simulink model "nominal_REALTIME"  (R2020b)
settings: Solver=FixedStepDiscrete  StartTime=0.0  StopTime=10.0  FixedStep=0.01  RelTol=1e-3  EnableMultiTasking=on
values from neighbouring files (symbols this model uses):
  denHw = [0.03 0 0 0]    [data_v2_500.mat]    (also in data_v6_nominaldrift500.mat)
  denLPFz = [1 -0.978482055734]    [data_v2_500.mat]    (also in data_v6_nominaldrift500.mat)
  drv =     [data_v2_500.mat]    (also in data_v6_nominaldrift500.mat)
  gbox =     [data_v2_500.mat]    (also in data_v6_nominaldrift500.mat)
  N_u = 0    [data_v2_500.mat]    (also in data_v6_nominaldrift500.mat)
  N_x = [1 0 0 0]    [data_v2_500.mat]    (also in data_v6_nominaldrift500.mat)
  numHw = [1 0 0 -1]    [data_v2_500.mat]    (also in data_v6_nominaldrift500.mat)
  numLPFz = [0.0215179442657 0]    [data_v2_500.mat]    (also in data_v6_nominaldrift500.mat)
  sens =     [data_v2_500.mat]    (also in data_v6_nominaldrift500.mat)
  Ts = 0.01    [data_v2_500.mat]    (also in data_v6_nominaldrift500.mat)
  wheel =     [data_v2_500.mat]    (also in data_v6_nominaldrift500.mat)
undefined symbols (not defined in the file or in its folder): C_gain, DiscIntNeverNeededParam, T
libraries: BalRobTbx_baselib x9
settings Model: SILPILModeSetting=veronly  ExtModeTrigDuration=2  Creator=utente  LastModifiedBy=saviangiul
settings OptimizationCC: EnhancedBackFolding=on  PassReuseOutputArgsAs=Individual arguments  ZeroExternalMemoryAtStartup=off  ZeroInternalMemoryAtStartup=off  MaxStackSize=64  OptimizeBlockOrder=speed  DifferentSizesBufferReuse=on  OptimizationCustomize=off  EfficientTunableParamExpr=on
settings DebuggingCC: ParameterTunabilityLossMsg=error
settings HardwareCC: ProdBitPerInt=16  ProdBitPerPointer=16  ProdBitPerSizeT=16  ProdBitPerPtrDiffT=16  ProdLargestAtomicFloat=None  ProdWordSize=8  ProdHWDeviceType=Atmel->AVR
settings SFSimCC: MATLABDynamicMemAlloc=off
settings RTWCC: Description=Embedded Coder  SystemTargetFile=ert.tlc  HardwareBoard=Arduino Mega 2560  TemplateMakefile=ert_default_tmf  Toolchain=Arduino AVR  BuildConfiguration=Faster Runs
settings CodeAppCC: ForceParamTrailComments=on  IgnoreCustomStorageClasses=off  OperatorAnnotations=on  SimulinkDataObjDesc=on  SFDataObjDesc=on  InsertBlockDesc=on
settings ERTTargetCC: SupportContinuousTime=on  SupportVariableSizeSignals=on  ExtModeStaticAllocSize=2048

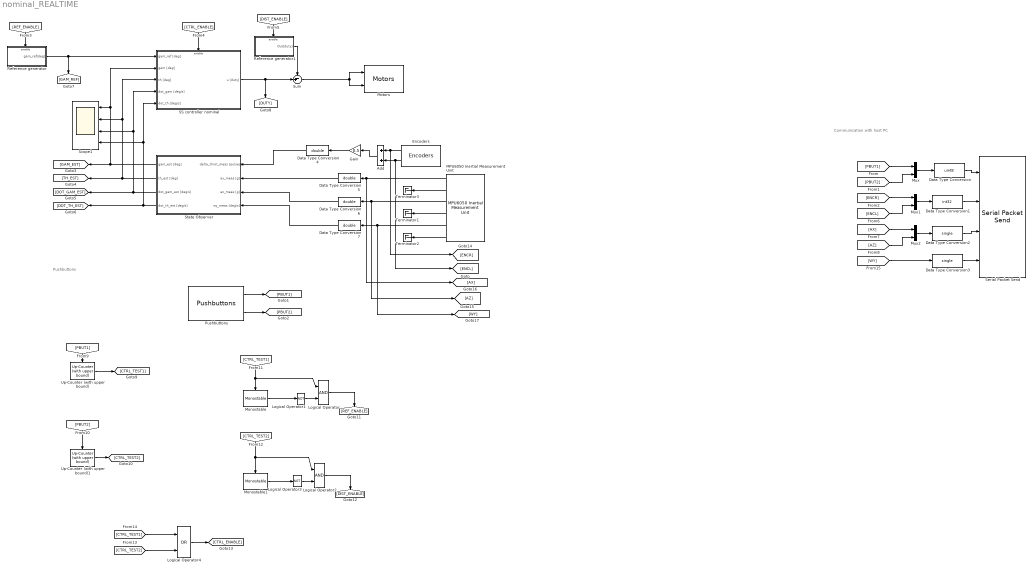
== system nominal_REALTIME ==
  note: Communication with host PC
  note: Pushbuttons
  Add : Sum
  Data Type Conversion : DataTypeConversion  OutDataTypeStr=uint8
  Data Type Conversion1 : DataTypeConversion  OutDataTypeStr=int32
  Data Type Conversion2 : DataTypeConversion  OutDataTypeStr=single
  Data Type Conversion3 : DataTypeConversion  OutDataTypeStr=single
  Data Type Conversion{4..7} (4 alike) : DataTypeConversion  OutDataTypeStr=double
  Encoders : BalRobTbx_baselib/Inputs/Encoders
      settings: SourceProductName=Balancing Robot Toolbox
  Gain : Gain  Gain=0.5
  Logical Operator : Logic  AllPortsSameDT=off  OutDataTypeStr=boolean
  Logical Operator1 : Logic  Operator=NOT  Inputs=1  AllPortsSameDT=off  OutDataTypeStr=boolean
  Logical Operator2 : Logic  AllPortsSameDT=off  OutDataTypeStr=boolean
  Logical Operator3 : Logic  Operator=NOT  Inputs=1  AllPortsSameDT=off  OutDataTypeStr=boolean
  Logical Operator4 : Logic  Operator=OR  AllPortsSameDT=off  OutDataTypeStr=boolean
  MPU6050 Inertial Measurement Unit : BalRobTbx_baselib/Inputs/MPU6050 Inertial Measurement Unit
      settings: SourceProductName=Balancing Robot Toolbox
  Monostable : BalRobTbx_baselib/Utilities/Monostable  Tp=1
      settings: SourceProductName=Balancing Robot Toolbox
  Monostable1 : BalRobTbx_baselib/Utilities/Monostable  Tp=1
      settings: SourceProductName=Balancing Robot Toolbox
  Motors : BalRobTbx_baselib/Outputs/Motors
      settings: SourceProductName=Balancing Robot Toolbox
  Mux : Mux  Inputs=2
  Mux1 : Mux  Inputs=2
  Mux2 : Mux  Inputs=2
  Pushbuttons : BalRobTbx_baselib/Inputs/Pushbuttons
      settings: SourceProductName=Balancing Robot Toolbox
  Reference generator : Subsystem
  Reference generator1 : Subsystem
  SS controller nominal : Subsystem
  Scope1 : Scope  NumInputPorts=4
  Serial Packet Send : BalRobTbx_baselib/Communication/Serial Packet Send  serialLinkOpt=Bluetooth  baudRateOpt=38400  waitHostTxCmd=on  txStartCmd=65  txStopCmd=66  packetSpec={'2*uint8', '2*int32', '2*single', 'single'}  cobsEncoded=on  nullTerminated=on  showEnablePort=off
      settings: SourceProductName=Balancing Robot Toolbox
  State Observer : Subsystem
  Sum : Sum  Inputs=-+|
  Terminator1 : Terminator
  Terminator2 : Terminator
  Terminator3 : Terminator
  Up-Counter (with upper bound) : BalRobTbx_baselib/Utilities/Up-Counter (with upper bound)  CMAX=10  C0=0
      settings: SourceProductName=Balancing Robot Toolbox
  Up-Counter (with upper bound)1 : BalRobTbx_baselib/Utilities/Up-Counter (with upper bound)  CMAX=10  C0=0
      settings: SourceProductName=Balancing Robot Toolbox
  wires:
  Reference generator/1(gam_ref[deg]) -> [GAM_REF], SS controller nominal/1(gam_ref [deg])
  Data Type Conversion4/1 -> State Observer/1("delta_throt_meas [pulses] ")
  State Observer/2(th_est [deg]) -> [TH_EST], SS controller nominal/3(th [deg]), Scope1/2
  Data Type Conversion6/1 -> State Observer/3("az_meas [g] ")
  Reference generator1/1(Out[duty]) -> Sum/1
  State Observer/1(gam_est [deg]) -> [GAM_EST], SS controller nominal/2(gam [deg]), Scope1/1
  SS controller nominal/1(u [duty]) -> [DUTY], Sum/2
  State Observer/4(dot_th_est [deg/s]) -> [DOT_TH_EST], SS controller nominal/5(dot_th [deg/s]), Scope1/4
  State Observer/3(dot_gam_est [deg/s]) -> [DOT_GAM_EST], SS controller nominal/4(dot_gam [deg/s]), Scope1/3
  Data Type Conversion7/1 -> State Observer/4(wy_meas [deg/s])
  [REF_ENABLE] -> Reference generator/Enable
  [CTRL_ENABLE] -> SS controller nominal/Enable
  [DIST_ENABLE] -> Reference generator1/Enable
  [CTRL_TEST1] -> Monostable/Enable, Logical Operator/1
  Logical Operator/1 -> [REF_ENABLE]
  Logical Operator1/1 -> Logical Operator/2
  Logical Operator3/1 -> Logical Operator2/2
  Logical Operator2/1 -> [DIST_ENABLE]
  [CTRL_TEST2] -> Logical Operator2/1, Monostable1/Enable
  [CTRL_TEST1] -> Logical Operator4/1
  [CTRL_TEST2] -> Logical Operator4/2
  Logical Operator4/1 -> [CTRL_ENABLE]
  Sum/1 -> Motors/2, Motors/1
  Pushbuttons/1 -> [PBUT1]
  Pushbuttons/2 -> [PBUT2]
  Monostable/1 -> Logical Operator1/1
  Monostable1/1 -> Logical Operator3/1
  Up-Counter (with upper bound)1/1 -> [CTRL_TEST2]
  [PBUT2] -> Up-Counter (with upper bound)1/Trigger
  [PBUT1] -> Up-Counter (with upper bound)/Trigger
  Up-Counter (with upper bound)/1 -> [CTRL_TEST1]
  [PBUT1] -> Mux/1
  [PBUT2] -> Mux/2
  [ENCR] -> Mux1/1
  [ENCL] -> Mux1/2
  [AX] -> Mux2/1
  [AZ] -> Mux2/2
  [WY] -> Data Type Conversion3/1
  Data Type Conversion3/1 -> Serial Packet Send/4
  Mux2/1 -> Data Type Conversion2/1
  Data Type Conversion2/1 -> Serial Packet Send/3
  Mux1/1 -> Data Type Conversion1/1
  Data Type Conversion1/1 -> Serial Packet Send/2
  Mux/1 -> Data Type Conversion/1
  Data Type Conversion/1 -> Serial Packet Send/1
  Encoders/2 -> Add/2, [ENCL]
  Gain/1 -> Data Type Conversion4/1
  MPU6050 Inertial Measurement Unit/3 -> [AZ], Data Type Conversion6/1
  MPU6050 Inertial Measurement Unit/5 -> [WY], Data Type Conversion7/1
  MPU6050 Inertial Measurement Unit/4 -> Terminator1/1
  Encoders/1 -> [ENCR], Add/1
  Add/1 -> Gain/1
  MPU6050 Inertial Measurement Unit/1 -> [AX], Data Type Conversion5/1
  MPU6050 Inertial Measurement Unit/2 -> Terminator3/1
  MPU6050 Inertial Measurement Unit/6 -> Terminator2/1
  Data Type Conversion5/1 -> State Observer/2("ax_meas [g] ")

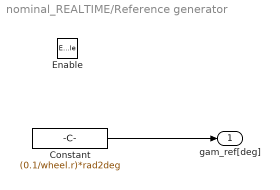
== system nominal_REALTIME/Reference generator ==
  Enable : EnablePort  StatesWhenEnabling=reset
  Constant : Constant  Value=(0.1/wheel.r)*rad2deg  SampleTime=0.01
  gam_ref[deg] : Outport  InitialOutput=[0]
  wires:
  Constant/1 -> gam_ref[deg]/1

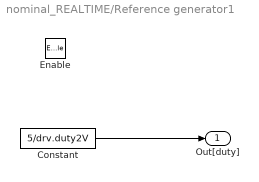
== system nominal_REALTIME/Reference generator1 ==
  Enable : EnablePort  StatesWhenEnabling=reset
  Constant : Constant  Value=5/drv.duty2V  SampleTime=0.01
  Out[duty] : Outport  InitialOutput=[0]
  wires:
  Constant/1 -> Out[duty]/1

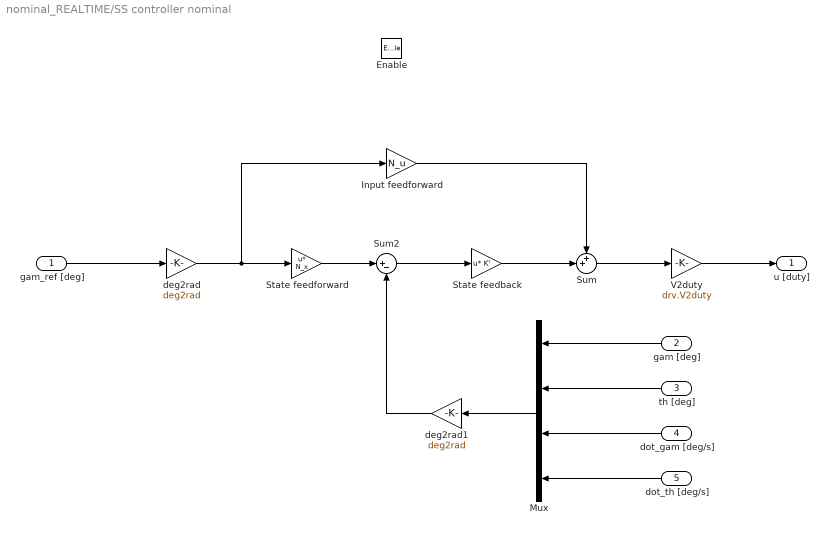
== system nominal_REALTIME/SS controller nominal ==
  gam_ref [deg] : Inport
  gam [deg] : Inport  Port=2
  th [deg] : Inport  Port=3
  dot_gam [deg/s] : Inport  Port=4
  dot_th [deg/s] : Inport  Port=5
  Enable : EnablePort  StatesWhenEnabling=reset
  Input feedforward : Gain  Gain=N_u
  Mux : Mux
  State feedback : Gain  Gain=K'  Multiplication=Matrix(u*K)
  "State feedforward\t" : Gain  Gain=N_x  Multiplication=Matrix(u*K)
  Sum : Sum  Inputs=++|
  Sum2 : Sum  Inputs=|+-
  V2duty : Gain  Gain=drv.V2duty
  deg2rad : Gain  Gain=deg2rad
  deg2rad1 : Gain  Gain=deg2rad
  u [duty] : Outport  InitialOutput=[0]
  wires:
  gam_ref [deg]/1 -> deg2rad/1
  deg2rad/1 -> Input feedforward/1, "State feedforward\t"/1
  State feedback/1 -> Sum/2
  "State feedforward\t"/1 -> Sum2/1
  Sum2/1 -> State feedback/1
  Input feedforward/1 -> Sum/1
  Sum/1 -> V2duty/1
  V2duty/1 -> u [duty]/1
  gam [deg]/1 -> Mux/1
  Mux/1 -> deg2rad1/1
  dot_gam [deg/s]/1 -> Mux/3
  th [deg]/1 -> Mux/2
  dot_th [deg/s]/1 -> Mux/4
  deg2rad1/1 -> Sum2/2

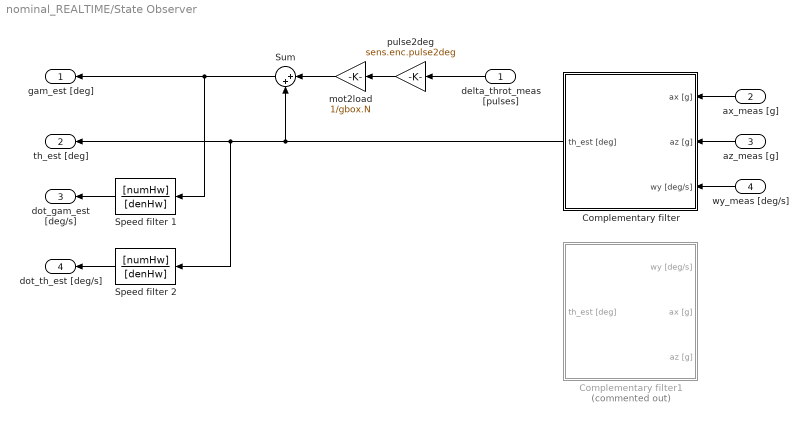
== system nominal_REALTIME/State Observer ==
  "delta_throt_meas [pulses] " : Inport
  "ax_meas [g] " : Inport  Port=2
  "az_meas [g] " : Inport  Port=3
  wy_meas [deg/s] : Inport  Port=4
  Complementary filter : Subsystem
  Complementary filter1 : Subsystem  Commented=on
  Speed filter 1 : DiscreteTransferFcn  Numerator=[numHw]  Denominator=[denHw]  SampleTime=Ts
  Speed filter 2 : DiscreteTransferFcn  Numerator=[numHw]  Denominator=[denHw]  SampleTime=Ts
  Sum : Sum  Inputs=|++
  mot2load : Gain  Gain=1/gbox.N
  pulse2deg : Gain  Gain=sens.enc.pulse2deg
  gam_est [deg] : Outport
  th_est [deg] : Outport  Port=2
  dot_gam_est [deg/s] : Outport  Port=3
  dot_th_est [deg/s] : Outport  Port=4
  wires:
  pulse2deg/1 -> mot2load/1
  "delta_throt_meas [pulses] "/1 -> pulse2deg/1
  mot2load/1 -> Sum/1
  Complementary filter/1("th_est [deg] ") -> Sum/2, Speed filter 2/1, th_est [deg]/1
  Sum/1 -> Speed filter 1/1, gam_est [deg]/1
  Speed filter 1/1 -> dot_gam_est [deg/s]/1
  Speed filter 2/1 -> dot_th_est [deg/s]/1
  "ax_meas [g] "/1 -> Complementary filter/1("ax [g] ")
  "az_meas [g] "/1 -> Complementary filter/2("az [g] ")
  wy_meas [deg/s]/1 -> Complementary filter/3(wy [deg/s])

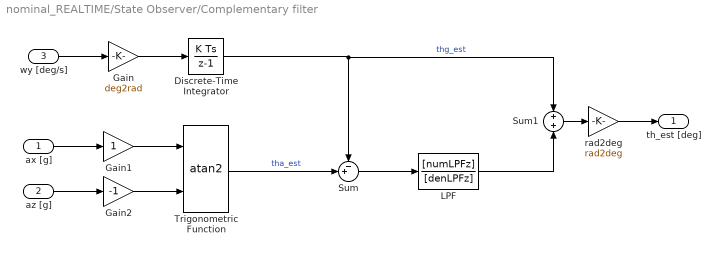
== system nominal_REALTIME/State Observer/Complementary filter ==
  "ax [g] " : Inport
  "az [g] " : Inport  Port=2
  wy [deg/s] : Inport  Port=3
  Discrete-Time Integrator : DiscreteIntegrator  gainval=1  SampleTime=Ts  ICPrevOutput=DiscIntNeverNeededParam  ICPrevScaledInput=DiscIntNeverNeededParam
  Gain : Gain  Gain=deg2rad
  Gain1 : Gain
  Gain2 : Gain  Gain=-1
  LPF : DiscreteTransferFcn  Numerator=[numLPFz]  Denominator=[denLPFz]  SampleTime=Ts
  Sum : Sum  Inputs=-+|
  Sum1 : Sum
  Trigonometric Function : Trigonometry  Operator=atan2
  rad2deg : Gain  Gain=rad2deg
  "th_est [deg] " : Outport
  wires:
  "az [g] "/1 -> Gain2/1
  "ax [g] "/1 -> Gain1/1
  wy [deg/s]/1 -> Gain/1
  Gain/1 -> Discrete-Time Integrator/1
  Gain2/1 -> Trigonometric Function/2
  Gain1/1 -> Trigonometric Function/1
  Trigonometric Function/1 -> Sum/2  "tha_est"
  Discrete-Time Integrator/1 -> Sum1/1, Sum/1  "thg_est"
  rad2deg/1 -> "th_est [deg] "/1
  Sum1/1 -> rad2deg/1
  Sum/1 -> LPF/1
  LPF/1 -> Sum1/2

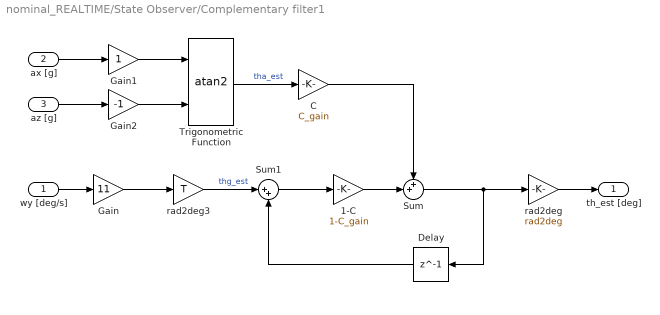
== system nominal_REALTIME/State Observer/Complementary filter1 ==
  wy [deg/s] : Inport
  "ax [g] " : Inport  Port=2
  "az [g] " : Inport  Port=3
  1-C : Gain  Gain=1-C_gain
  C : Gain  Gain=C_gain
  Delay : Delay  DelayLength=1
  Gain : Gain  Gain=11
  Gain1 : Gain
  Gain2 : Gain  Gain=-1
  Sum : Sum  Inputs=++|
  Sum1 : Sum  Inputs=|++
  Trigonometric Function : Trigonometry  Operator=atan2
  rad2deg : Gain  Gain=rad2deg
  rad2deg3 : Gain  Gain=T
  "th_est [deg] " : Outport
  wires:
  "az [g] "/1 -> Gain2/1
  "ax [g] "/1 -> Gain1/1
  wy [deg/s]/1 -> Gain/1
  Gain/1 -> rad2deg3/1
  Gain2/1 -> Trigonometric Function/2
  Gain1/1 -> Trigonometric Function/1
  rad2deg/1 -> "th_est [deg] "/1
  Trigonometric Function/1 -> C/1  "tha_est"
  C/1 -> Sum/1
  1-C/1 -> Sum/2
  Sum/1 -> Delay/1, rad2deg/1
  Delay/1 -> Sum1/2
  rad2deg3/1 -> Sum1/1  "thg_est"
  Sum1/1 -> 1-C/1
